simulink model "Dynamic_PID_Cascaded"  (R2017b)
settings: Solver=ode5  StartTime=0.0  StopTime=7.1423  FixedStep=0.02  RelTol=1e-3
settings Model: Creator=Admin  LastModifiedBy=Admin
settings CodeAppCC: StateflowObjectComments=on

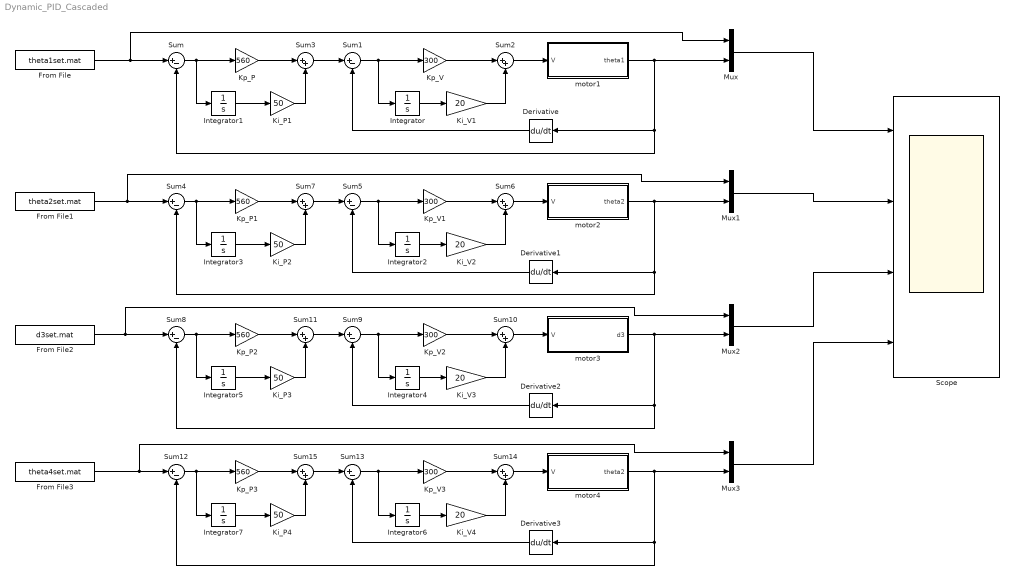
== system Dynamic_PID_Cascaded ==
  Derivative{,1..3} (4 alike) : Derivative
  From File : FromFile  FileName=theta1set.mat
  From File1 : FromFile  FileName=theta2set.mat
  From File2 : FromFile  FileName=d3set.mat
  From File3 : FromFile  FileName=theta4set.mat
  Integrator{,1..7} (8 alike) : Integrator
  Ki_P{1..4} (4 alike) : Gain  Gain=50
  Ki_V{1..4} (4 alike) : Gain  Gain=20
  Kp_P{,1..3} (4 alike) : Gain  Gain=560
  Kp_V{,1..3} (4 alike) : Gain  Gain=300
  Mux{,1..3} (4 alike) : Mux  Inputs=2
  Scope : Scope  NumInputPorts=4
  Sum{,1,4..5,8..9,12..13} (8 alike) : Sum  Inputs=|+-
  Sum{2..3,6..7,10..11,14..15} (8 alike) : Sum  Inputs=|++
  motor1 : Subsystem  mask{Ki=0.1, Kb=0.1, L=0.5, R=2, Jeff=0.02, Beff=0.2, N=200}
  motor2 : Subsystem  mask{Ki=0.1, Kb=0.1, L=0.5, R=2, Jeff=0.02, Beff=0.2, N=100}
  motor3 : Subsystem  mask{Ki=0.1, Kb=0.1, L=0.5, R=2, Jeff=0.02, Beff=0.2, N=100}
  motor4 : Subsystem  mask{Ki=0.1, Kb=0.1, L=0.5, R=2, Jeff=0.02, Beff=0.2, N=100}
  wires:
  motor1/1(theta1) -> Mux/2, Sum/2, Derivative/1
  Sum1/1 -> Integrator/1, Kp_V/1
  Sum2/1 -> motor1/1(V)
  Integrator/1 -> Ki_V1/1
  Kp_V/1 -> Sum2/1
  Ki_V1/1 -> Sum2/2
  Derivative/1 -> Sum1/2
  From File/1 -> Mux/1, Sum/1
  Sum/1 -> Integrator1/1, Kp_P/1
  Sum3/1 -> Sum1/1
  Integrator1/1 -> Ki_P1/1
  Ki_P1/1 -> Sum3/2
  Kp_P/1 -> Sum3/1
  motor2/1(theta2) -> Mux1/2, Sum4/2, Derivative1/1
  Ki_P2/1 -> Sum7/2
  Kp_P1/1 -> Sum7/1
  Integrator3/1 -> Ki_P2/1
  Sum7/1 -> Sum5/1
  Sum4/1 -> Integrator3/1, Kp_P1/1
  From File1/1 -> Mux1/1, Sum4/1
  Sum6/1 -> motor2/1(V)
  Sum5/1 -> Integrator2/1, Kp_V1/1
  Integrator2/1 -> Ki_V2/1
  Ki_V2/1 -> Sum6/2
  Kp_V1/1 -> Sum6/1
  Derivative1/1 -> Sum5/2
  Integrator4/1 -> Ki_V3/1
  Derivative2/1 -> Sum9/2
  Kp_V2/1 -> Sum10/1
  Kp_P2/1 -> Sum11/1
  From File2/1 -> Mux2/1, Sum8/1
  Ki_V3/1 -> Sum10/2
  Sum8/1 -> Integrator5/1, Kp_P2/1
  Ki_P3/1 -> Sum11/2
  Sum11/1 -> Sum9/1
  motor3/1(d3) -> Mux2/2, Sum8/2, Derivative2/1
  Sum10/1 -> motor3/1(V)
  Sum9/1 -> Integrator4/1, Kp_V2/1
  Integrator5/1 -> Ki_P3/1
  Integrator6/1 -> Ki_V4/1
  Derivative3/1 -> Sum13/2
  Kp_V3/1 -> Sum14/1
  Kp_P3/1 -> Sum15/1
  From File3/1 -> Mux3/1, Sum12/1
  Ki_V4/1 -> Sum14/2
  Sum12/1 -> Integrator7/1, Kp_P3/1
  Ki_P4/1 -> Sum15/2
  Sum15/1 -> Sum13/1
  motor4/1(theta2) -> Mux3/2, Sum12/2, Derivative3/1
  Sum14/1 -> motor4/1(V)
  Sum13/1 -> Integrator6/1, Kp_V3/1
  Integrator7/1 -> Ki_P4/1
  Mux/1 -> Scope/1
  Mux1/1 -> Scope/2
  Mux2/1 -> Scope/3
  Mux3/1 -> Scope/4

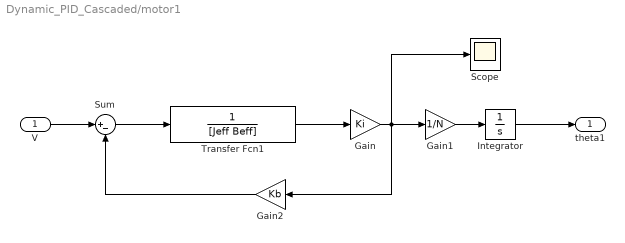
== system Dynamic_PID_Cascaded/motor1 ==
  V : Inport
  Gain : Gain  Gain=Ki
  Gain1 : Gain  Gain=1/N
  Gain2 : Gain  Gain=Kb
  Integrator : Integrator
  Scope : Scope
  Sum : Sum  Inputs=|+-
  Transfer Fcn1 : TransferFcn  Denominator=[Jeff Beff]
  theta1 : Outport
  wires:
  Transfer Fcn1/1 -> Gain/1
  Gain2/1 -> Sum/2
  V/1 -> Sum/1
  Sum/1 -> Transfer Fcn1/1
  Gain/1 -> Gain1/1, Gain2/1, Scope/1
  Gain1/1 -> Integrator/1
  Integrator/1 -> theta1/1

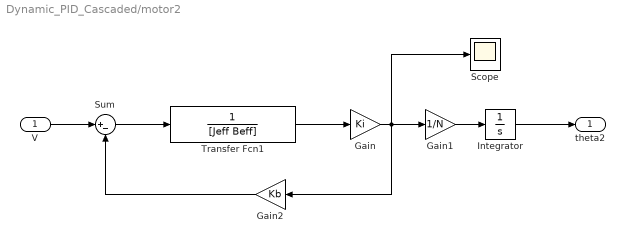
== system Dynamic_PID_Cascaded/motor2 ==
  V : Inport
  Gain : Gain  Gain=Ki
  Gain1 : Gain  Gain=1/N
  Gain2 : Gain  Gain=Kb
  Integrator : Integrator
  Scope : Scope
  Sum : Sum  Inputs=|+-
  Transfer Fcn1 : TransferFcn  Denominator=[Jeff Beff]
  theta2 : Outport
  wires:
  Transfer Fcn1/1 -> Gain/1
  Gain2/1 -> Sum/2
  V/1 -> Sum/1
  Sum/1 -> Transfer Fcn1/1
  Gain/1 -> Gain1/1, Gain2/1, Scope/1
  Gain1/1 -> Integrator/1
  Integrator/1 -> theta2/1

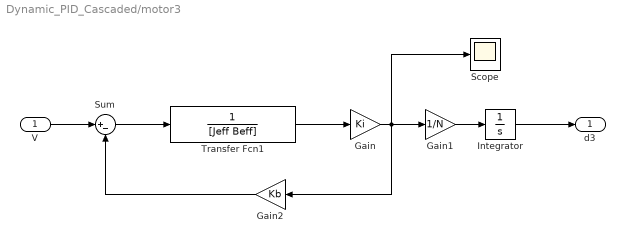
== system Dynamic_PID_Cascaded/motor3 ==
  V : Inport
  Gain : Gain  Gain=Ki
  Gain1 : Gain  Gain=1/N
  Gain2 : Gain  Gain=Kb
  Integrator : Integrator
  Scope : Scope
  Sum : Sum  Inputs=|+-
  Transfer Fcn1 : TransferFcn  Denominator=[Jeff Beff]
  d3 : Outport
  wires:
  Transfer Fcn1/1 -> Gain/1
  Gain2/1 -> Sum/2
  V/1 -> Sum/1
  Sum/1 -> Transfer Fcn1/1
  Gain/1 -> Gain1/1, Gain2/1, Scope/1
  Gain1/1 -> Integrator/1
  Integrator/1 -> d3/1

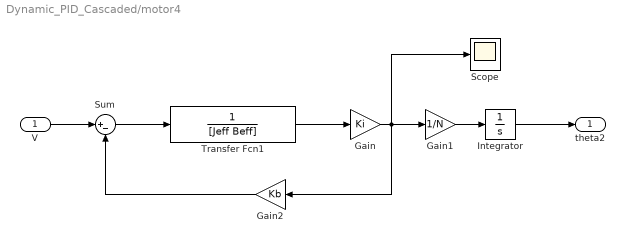
== system Dynamic_PID_Cascaded/motor4 ==
  V : Inport
  Gain : Gain  Gain=Ki
  Gain1 : Gain  Gain=1/N
  Gain2 : Gain  Gain=Kb
  Integrator : Integrator
  Scope : Scope
  Sum : Sum  Inputs=|+-
  Transfer Fcn1 : TransferFcn  Denominator=[Jeff Beff]
  theta2 : Outport
  wires:
  Transfer Fcn1/1 -> Gain/1
  Gain2/1 -> Sum/2
  V/1 -> Sum/1
  Sum/1 -> Transfer Fcn1/1
  Gain/1 -> Gain1/1, Gain2/1, Scope/1
  Gain1/1 -> Integrator/1
  Integrator/1 -> theta2/1
